simulink library "variableFlowProfileCalculationYZ_ul"  (R2018b)
settings: Solver=VariableStepAuto  StartTime=0.0  StopTime=10.0  RelTol=1e-3
libraries: dspmtrx3 x6, Dynamic_2D_Lookup_Table x3
settings Model: Creator=James Reed  LastModifiedBy=James Reed

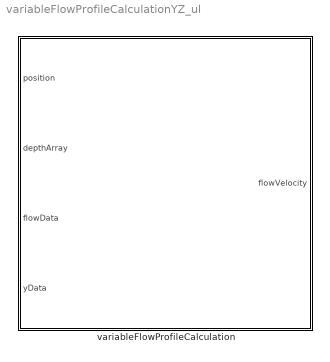
== system variableFlowProfileCalculationYZ_ul ==
  variableFlowProfileCalculation : Subsystem

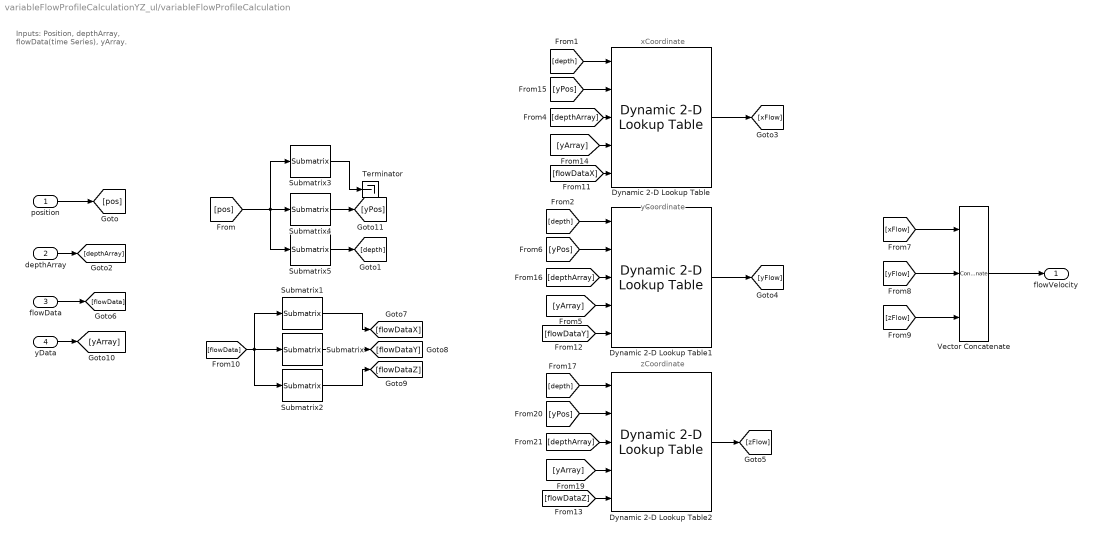
== system variableFlowProfileCalculationYZ_ul/variableFlowProfileCalculation ==
  note: Inputs: Position, depthArray,
      | flowData(time Series), yArray.
  note: xCoordinate
  note: zCoordinate
  note: yCoordinate
  "position " : Inport
  "depthArray " : Inport  Port=2
  "flowData " : Inport  Port=3
  "yData " : Inport  Port=4
  Dynamic 2-D Lookup Table : Dynamic_2D_Lookup_Table/Dynamic 2-D Lookup Table
  Dynamic 2-D Lookup Table1 : Dynamic_2D_Lookup_Table/Dynamic 2-D Lookup Table
  Dynamic 2-D Lookup Table2 : Dynamic_2D_Lookup_Table/Dynamic 2-D Lookup Table
  Submatrix : dspmtrx3/Submatrix  RowSpan=One row  RowStartMode=Middle  RowStartIndex=1  RowEndMode=Last  RowEndIndex=1  ColSpan=All columns  ColStartMode=First  ColStartIndex=1  ColEndMode=Last  ColEndIndex=1
  Submatrix{1,3..5} (4 alike) : dspmtrx3/Submatrix  RowSpan=One row  RowStartMode=First  RowStartIndex=1  RowEndMode=Last  RowEndIndex=1  ColSpan=All columns  ColStartMode=First  ColStartIndex=1  ColEndMode=Last  ColEndIndex=1
  Submatrix2 : dspmtrx3/Submatrix  RowSpan=One row  RowStartMode=Last  RowStartIndex=1  RowEndMode=Last  RowEndIndex=1  ColSpan=All columns  ColStartMode=First  ColStartIndex=1  ColEndMode=Last  ColEndIndex=1
  Terminator : Terminator
  Vector Concatenate : Concatenate  NumInputs=3  Mode=Multidimensional array
  "flowVelocity " : Outport
  wires:
  Submatrix2/1 -> [flowDataZ]
  [pos] -> Submatrix3/1, Submatrix5/1, Submatrix4/1
  [depthArray] -> Dynamic 2-D Lookup Table/3
  Dynamic 2-D Lookup Table2/1 -> [zFlow]
  Dynamic 2-D Lookup Table/1 -> [xFlow]
  Submatrix1/1 -> [flowDataX]
  Submatrix3/1 -> Terminator/1
  [flowData] -> Submatrix/1, Submatrix1/1, Submatrix2/1
  "depthArray "/1 -> [depthArray]
  Submatrix/1 -> [flowDataY]
  Submatrix5/1 -> [depth]
  "flowData "/1 -> [flowData]
  [depth] -> Dynamic 2-D Lookup Table/1
  [yFlow] -> Vector Concatenate/2
  [flowDataX] -> Dynamic 2-D Lookup Table/5
  [xFlow] -> Vector Concatenate/1
  Submatrix4/1 -> [yPos]
  Vector Concatenate/1 -> "flowVelocity "/1
  "position "/1 -> [pos]
  [zFlow] -> Vector Concatenate/3
  "yData "/1 -> [yArray]
  [yArray] -> Dynamic 2-D Lookup Table/4
  [yPos] -> Dynamic 2-D Lookup Table/2
  [depth] -> Dynamic 2-D Lookup Table1/1
  [yPos] -> Dynamic 2-D Lookup Table1/2
  [yArray] -> Dynamic 2-D Lookup Table1/4
  [depthArray] -> Dynamic 2-D Lookup Table1/3
  [flowDataZ] -> Dynamic 2-D Lookup Table2/5
  [depth] -> Dynamic 2-D Lookup Table2/1
  [yPos] -> Dynamic 2-D Lookup Table2/2
  [yArray] -> Dynamic 2-D Lookup Table2/4
  [depthArray] -> Dynamic 2-D Lookup Table2/3
  Dynamic 2-D Lookup Table1/1 -> [yFlow]
  [flowDataY] -> Dynamic 2-D Lookup Table1/5
